simulink model "MC_SinglePulseN6"  (R2014b)
settings: Solver=FixedStepDiscrete  StartTime=0.0  StopTime=300  FixedStep=1.0  RelTol=1e-3
undefined symbols (not defined in the file or in its folder): delTimes
libraries: BlockLib x21, dspsrcs4 x1
settings Model: Creator=lstmarie  LastModifiedBy=Alexander
settings DebuggingCC: UnderspecifiedInitializationDetection=Classic  MergeDetectMultiDrivingBlocksExec=none

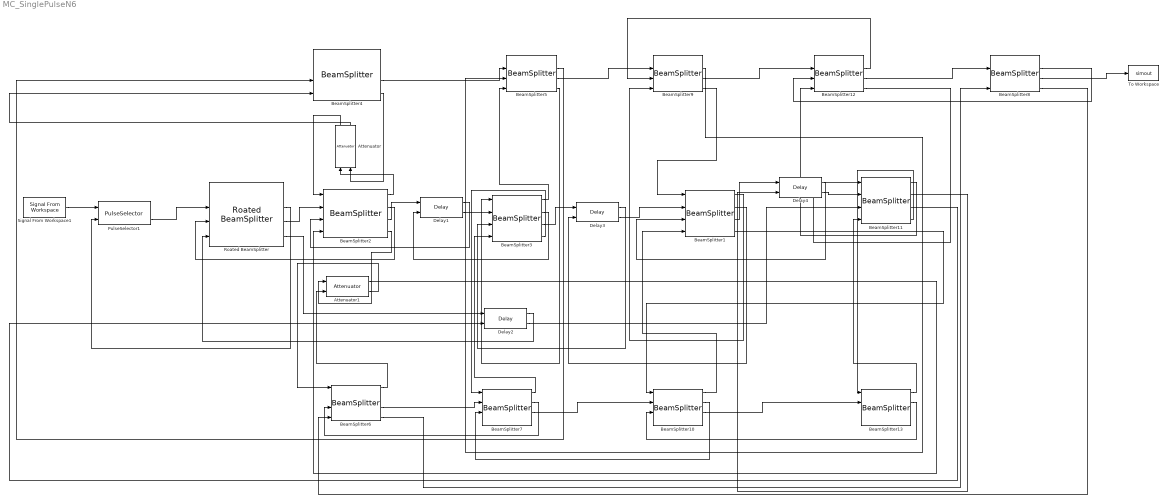
== system MC_SinglePulseN6 ==
  Attenuator : BlockLib/Attenuator  AttnFactor=0.5
  Attenuator1 : BlockLib/Attenuator  AttnFactor=0.5
  BeamSplitter{1..13} (13 alike) : BlockLib/BeamSplitter  Transmittance=0.50  Reflectance=0.50  Ghost=0.01  BackReflectance=0.001
  Delay1 : BlockLib/Delay  DelayAmt=delTimes(1)
  Delay2 : BlockLib/Delay  DelayAmt=delTimes(4)
  Delay3 : BlockLib/Delay  DelayAmt=delTimes(2)
  Delay4 : BlockLib/Delay  DelayAmt=delTimes(3)
  PulseSelector1 : BlockLib/PulseSelector  PCTimings=PCTimings1  ControlPowers=CP1
  Roated BeamSplitter : BlockLib/Roated BeamSplitter  Transmittance=0.5  Reflectance=0.5  Ghost=0.01  BackReflectance=0.001
  Signal From Workspace1 : dspsrcs4/Signal From Workspace  X=inputsignal  Ts=1  nsamps=1  OutputAfterFinalValue=Setting to zero  ignoreOrWarnInputAndFrameLengths=off
  To Workspace : ToWorkspace  VariableName=simout  SaveFormat=Timeseries  SampleTime=-1
  wires:
  Signal From Workspace1/1 -> PulseSelector1/1
  Roated BeamSplitter/4 -> Delay2/1
  Delay2/1 -> Roated BeamSplitter/4
  BeamSplitter2/2 -> Roated BeamSplitter/3
  Roated BeamSplitter/2 -> PulseSelector1/2
  BeamSplitter2/3 -> Delay1/1
  Delay1/1 -> BeamSplitter2/3
  BeamSplitter4/3 -> BeamSplitter5/2
  BeamSplitter5/2 -> BeamSplitter4/3
  BeamSplitter6/3 -> BeamSplitter7/2
  BeamSplitter7/2 -> BeamSplitter6/3
  Delay1/2 -> BeamSplitter3/2
  BeamSplitter3/2 -> Delay1/2
  BeamSplitter3/3 -> Delay3/1
  Delay3/1 -> BeamSplitter3/3
  BeamSplitter3/1 -> BeamSplitter5/4
  BeamSplitter5/4 -> BeamSplitter3/1
  BeamSplitter7/1 -> BeamSplitter3/4
  BeamSplitter3/4 -> BeamSplitter7/1
  BeamSplitter9/2 -> BeamSplitter5/3
  BeamSplitter5/3 -> BeamSplitter9/2
  BeamSplitter7/3 -> BeamSplitter10/2
  BeamSplitter10/2 -> BeamSplitter7/3
  BeamSplitter1/2 -> Delay3/2
  Delay3/2 -> BeamSplitter1/2
  BeamSplitter1/4 -> BeamSplitter10/1
  BeamSplitter10/1 -> BeamSplitter1/4
  BeamSplitter9/4 -> BeamSplitter1/1
  BeamSplitter1/1 -> BeamSplitter9/4
  PulseSelector1/2 -> Roated BeamSplitter/2
  Roated BeamSplitter/3 -> BeamSplitter2/2
  BeamSplitter8/3 -> To Workspace/1
  BeamSplitter2/1 -> Attenuator/1
  BeamSplitter4/4 -> Attenuator/2
  BeamSplitter2/4 -> Attenuator1/1
  Attenuator1/2 -> BeamSplitter6/1
  Attenuator/2 -> BeamSplitter4/4
  Attenuator/1 -> BeamSplitter2/1
  BeamSplitter6/1 -> Attenuator1/2
  Attenuator1/1 -> BeamSplitter2/4
  BeamSplitter13/2 -> BeamSplitter10/3
  BeamSplitter10/3 -> BeamSplitter13/2
  BeamSplitter13/1 -> BeamSplitter11/4
  BeamSplitter11/4 -> BeamSplitter13/1
  BeamSplitter12/2 -> BeamSplitter9/3
  BeamSplitter11/1 -> BeamSplitter12/4
  BeamSplitter12/4 -> BeamSplitter11/1
  BeamSplitter9/3 -> BeamSplitter12/2
  BeamSplitter8/2 -> BeamSplitter12/3
  BeamSplitter12/3 -> BeamSplitter8/2
  BeamSplitter11/3 -> Delay2/2
  Delay2/2 -> BeamSplitter11/3
  BeamSplitter6/4 -> BeamSplitter8/4
  BeamSplitter8/4 -> BeamSplitter6/4
  BeamSplitter1/3 -> Delay4/1
  Delay4/2 -> BeamSplitter11/2
  BeamSplitter11/2 -> Delay4/2
  Delay4/1 -> BeamSplitter1/3
